simulink model "conSys_2robots_2_vR2014a"  (Simulink 8.3)
settings: Solver=FixedStepDiscrete  StartTime=0.0  StopTime=200  FixedStep=Ts  RelTol=1e-3
values from neighbouring files (symbols this model uses):
  ck = double(max(abs([par.q0_r1;par.q0_r2] - [par.q0r_r1;par.q0r_r2]))*20/7000 + 6)    [startUp_conSys_2robots_1_vGPU_vR2014a.m]    (also in startUp_conSys_2robots_1_vR2014a.m = max(abs([par.q0_r1;par.q0_r2] - [par.q0r_r1;par.q0r_r2]))*20; startUp_conSys_2robots_2_vR2014a.m = max(abs([par.q0_r1;par.q0_r2] - [par.q0r_r1;par.q0r_r2]))*20; startUp_conSys_2robots_3_vR2014a.m = max(abs([par.q0_r1;par.q0_r2] - [par.q0r_r1;par.q0r_r2]))*20; startUp_conSys_2robots_4_vR2014a.m = max(abs([par.q0_r1;par.q0_r2] - [par.q0r_r1;par.q0r_r2]))*20)
  d_0 = 2000    [startUp_conSys_2robots_1_vGPU_vR2014a.m]    (also in startUp_conSys_2robots_1_vR2014a.m = 200; startUp_conSys_2robots_2_vR2014a.m = 200; startUp_conSys_2robots_3_vR2014a.m; startUp_conSys_2robots_4_vR2014a.m = 200)
  do1r_0 = dthc_0 + dph1_0    (= 0.2)    [startUp_conSys_2robots_1_vGPU_vR2014a.m]    (also in startUp_conSys_2robots_1_vR2014a.m = 0; startUp_conSys_2robots_2_vR2014a.m = 0; startUp_conSys_2robots_3_vR2014a.m = 0; startUp_conSys_2robots_4_vR2014a.m = 0)
  do2r_0 = dthc_0 + dph2_0    (= -0.2)    [startUp_conSys_2robots_1_vGPU_vR2014a.m]    (also in startUp_conSys_2robots_1_vR2014a.m = 0; startUp_conSys_2robots_2_vR2014a.m = 0; startUp_conSys_2robots_3_vR2014a.m = 0; startUp_conSys_2robots_4_vR2014a.m = 0)
  dx1r_0 = dxc_0 + sin(thc_0)*dd_0 + d_0*cos(thc_0)*dthc_0    [startUp_conSys_2robots_1_vGPU_vR2014a.m]    (also in startUp_conSys_2robots_1_vR2014a.m; startUp_conSys_2robots_2_vR2014a.m; startUp_conSys_2robots_3_vR2014a.m; startUp_conSys_2robots_4_vR2014a.m)
  dx2r_0 = dxc_0 - sin(thc_0)*dd_0 - d_0*cos(thc_0)*dthc_0    [startUp_conSys_2robots_1_vGPU_vR2014a.m]    (also in startUp_conSys_2robots_1_vR2014a.m; startUp_conSys_2robots_2_vR2014a.m; startUp_conSys_2robots_3_vR2014a.m; startUp_conSys_2robots_4_vR2014a.m)
  dy1r_0 = dyc_0 + cos(thc_0)*dd_0 - d_0*sin(thc_0)*dthc_0    [startUp_conSys_2robots_1_vGPU_vR2014a.m]    (also in startUp_conSys_2robots_1_vR2014a.m; startUp_conSys_2robots_2_vR2014a.m; startUp_conSys_2robots_3_vR2014a.m; startUp_conSys_2robots_4_vR2014a.m)
  dy2r_0 = dyc_0 - cos(thc_0)*dd_0 + d_0*sin(thc_0)*dthc_0    [startUp_conSys_2robots_1_vGPU_vR2014a.m]    (also in startUp_conSys_2robots_1_vR2014a.m; startUp_conSys_2robots_2_vR2014a.m; startUp_conSys_2robots_3_vR2014a.m; startUp_conSys_2robots_4_vR2014a.m)
  o1r_0 = pi/2 - thc_0    (= 0)    [startUp_conSys_2robots_1_vGPU_vR2014a.m]    (also in startUp_conSys_2robots_1_vR2014a.m = pi/2 - thc_0; startUp_conSys_2robots_2_vR2014a.m = pi/2 - thc_0; startUp_conSys_2robots_3_vR2014a.m; startUp_conSys_2robots_4_vR2014a.m = th1_0)
  o2r_0 = pi/2 - thc_0    (= 0)    [startUp_conSys_2robots_1_vGPU_vR2014a.m]    (also in startUp_conSys_2robots_1_vR2014a.m = pi/2 - thc_0; startUp_conSys_2robots_2_vR2014a.m = pi/2 - thc_0; startUp_conSys_2robots_3_vR2014a.m; startUp_conSys_2robots_4_vR2014a.m = th2_0)
  thc_0 = pi/2    (= 1.57079632679)    [startUp_conSys_2robots_1_vGPU_vR2014a.m]    (also in startUp_conSys_2robots_1_vR2014a.m = atan2(1/25,1/12.5) + pi/2; startUp_conSys_2robots_2_vR2014a.m = atan2(1/25,1/12.5) + pi/2; startUp_conSys_2robots_3_vR2014a.m; startUp_conSys_2robots_4_vR2014a.m = atan2(1/25,1/12.5) + pi/2)
  Ts = 1/200    (= 0.005)    [startUp_conSys_2robots_1_vGPU_vR2014a.m]    (also in startUp_conSys_2robots_1_vR2014a.m = 0.0125; startUp_conSys_2robots_2_vR2014a.m = 0.01; startUp_conSys_2robots_3_vR2014a.m; startUp_conSys_2robots_4_vR2014a.m)
  x1_0 = 12000    [startUp_conSys_2robots_1_vGPU_vR2014a.m]    (also in startUp_conSys_2robots_1_vR2014a.m = 13178.9; startUp_conSys_2robots_2_vR2014a.m = 13178.9; startUp_conSys_2robots_3_vR2014a.m; startUp_conSys_2robots_4_vR2014a.m = 13178.9)
  x2_0 = 8000    [startUp_conSys_2robots_1_vGPU_vR2014a.m]    (also in startUp_conSys_2robots_1_vR2014a.m = 12821.1; startUp_conSys_2robots_2_vR2014a.m = 12821.1; startUp_conSys_2robots_3_vR2014a.m; startUp_conSys_2robots_4_vR2014a.m = 12821.1)
  xc_0 = 10000    [startUp_conSys_2robots_1_vGPU_vR2014a.m]    (also in startUp_conSys_2robots_1_vR2014a.m = 13000; startUp_conSys_2robots_2_vR2014a.m = 13000; startUp_conSys_2robots_3_vR2014a.m; startUp_conSys_2robots_4_vR2014a.m = 13000)
  y1_0 = 10000    [startUp_conSys_2robots_1_vGPU_vR2014a.m]    (also in startUp_conSys_2robots_1_vR2014a.m = 12910.6; startUp_conSys_2robots_2_vR2014a.m = 12910.6; startUp_conSys_2robots_3_vR2014a.m; startUp_conSys_2robots_4_vR2014a.m = 12910.6)
  y2_0 = 10000    [startUp_conSys_2robots_1_vGPU_vR2014a.m]    (also in startUp_conSys_2robots_1_vR2014a.m = 13089.4; startUp_conSys_2robots_2_vR2014a.m = 13089.4; startUp_conSys_2robots_3_vR2014a.m; startUp_conSys_2robots_4_vR2014a.m = 13089.4)
  yc_0 = 10000    [startUp_conSys_2robots_1_vGPU_vR2014a.m]    (also in startUp_conSys_2robots_1_vR2014a.m = 13000; startUp_conSys_2robots_2_vR2014a.m = 13000; startUp_conSys_2robots_3_vR2014a.m; startUp_conSys_2robots_4_vR2014a.m = 13000)
undefined symbols (not defined in the file or in its folder): absoluteAngle01_vR2014a, absoluteAngle02_vR2014a, absoluteAngle03_vR2014a, absoluteAngle04_vR2014a, absoluteAngle05_vR2014a, absoluteAngle06_vR2014a, absoluteAngle07_vR2014a, DiscIntNeverNeededParam
undefined symbols (not defined in the file): ADAMS_cwd, ADAMS_exec, ADAMS_host, ADAMS_init, ADAMS_inputs, ADAMS_outputs, ADAMS_prefix, ADAMS_static, ADAMS_sysdir
libraries: simulink x18, cstblocks x1
(part 2 of 2)

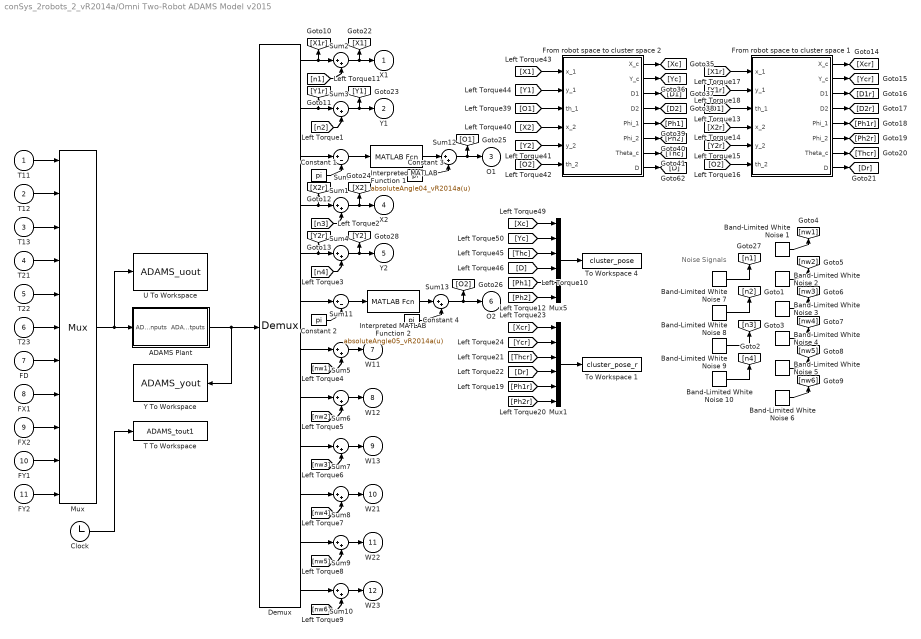
== system conSys_2robots_2_vR2014a/Omni Two-Robot ADAMS Model v2015 ==
  note: Noise Signals
  T11 : Inport
  T12 : Inport  Port=2
  T13 : Inport  Port=3
  T21 : Inport  Port=4
  T22 : Inport  Port=5
  T23 : Inport  Port=6
  FD : Inport  Port=7
  FX1 : Inport  Port=8
  FX2 : Inport  Port=9
  FY1 : Inport  Port=10
  FY2 : Inport  Port=11
  ADAMS Plant : Subsystem  LoadFcn=|  InitFcn=clear mex  mask(Adams Plant){exevie=ADAMS_sysdir, nam_in=ADAMS_inputs, namout=ADAMS_outputs, nampre=ADAMS_prefix, outfil=ADAMS_prefix, exesol=ADAMS_exec, stat=ADAMS_static, inicmd=[ADAMS_init], exetyp=C++, comtyp=PIPE(DDE), workdir=ADAMS_cwd, ada_host=ADAMS_host, modani=batch, modsim=discrete, dft=no, simulink_lead_cosim=yes, pin_interp_order=0, pout_extrap_order=0, pin_extrap_order=0, pout_interp_order=0, dt_out=Ts, o_rate=1, more=off}
      | %check based on dialog box setting for when setting by popup menu                                             
      | if exist('ADAMS_solver_type')                                                                                 
      |   if strcmp(ADAMS_solver_type,'C++')                                                                          
      |     set_param(gcb,'exetyp','C++');                                                                            
      |   else                                                                                                        
      |     set_param(gcb,'exetyp','Fortran');                                                                        
      |   end                                                                                                         
      | else                                                                                                          
      |   set_param(gcb,'exetyp','C++');                                                                              
      | end                                                                                                           
      | %set the mode if using acar_solver                                                                            
      | %REQUIRED HERE BECAUSE BELOW CAUSES MDLTERMINATE TO BE CALLED 2 TIMES IN MIDDLE OF SIMULATION WHEN SET IN MASK
      |                                                                                                               
      | %enable the direct feedthrough, sim mode, anim mode parameters by default                                     
      |                                                                                                               
      | if exist('set_some_params_states')                                                                            
      |                                                                                                               
      |   set_some_params_states({'dft','modsim','modani'},{'on','on','on'},'MaskEnables',gcb)                        
      |   %turn on direct feedthrough option                                                                          
      |   set_some_params_states({'dft'},{'on'},'MaskVisibilities',gcb)                                               
      |                                                                                                               
      |  end                                                                                                          
      |                                                                                                               
      |                                                                                                               
      | if exist('ADAMS_exec')                                                                                        
      |   if and(strcmp(get_param(gcb,'exesol'),'ADAMS_exec'),strcmp(ADAMS_exec,'acar_solver'))                       
      |     %set the sim mode to discrete -- only supported mode                                                      
      |     set_param(gcb,'modsim','discrete')                                                                        
      |      %turn off direct feedthrough option                                                                      
      |      set_some_params_states({'dft'},{'off'},'MaskVisibilities',gcb)                                           
      |     %set the animation mode to batch -- only supported mode                                                   
      |     set_param(gcb,'modani','batch')                                                                           
      |     %disable the direct feedthrough, sim mode, anim mode parameters                                           
      |     set_some_params_states({'modsim','modani'},{'off','off'},'MaskEnables',gcb)                               
      |   end                                                                                                         
      | end
      mask prompts: exevie "Adams install directory"; nam_in "Adams/View input names"; namout "Adams/View output names"; nampre "Adams model file prefix"; outfil "Output files prefix (opt.: if blank - no output)"; exesol "User executable (opt.: if blank - use standard)"; stat "Initial static simulation flag"; inicmd "Initialization commands"; exetyp "Adams/Solver type"; comtyp "Interprocess option"; workdir "Adams working directory"; ada_host "Adams host"; modani "Animation mode"; modsim "Simulation mode"; dft "Direct feedthrough"; simulink_lead_cosim "Discrete Computational Order - Simulink Leads Adams"; pin_interp_order "Plant input interpolation order"; pout_extrap_order "Plant output extrapolation order"; pin_extrap_order "Plant input extrapolation order"; pout_interp_order "Plant output interpolation order"; dt_out "Communication interval"; o_rate "Number of communications per output step"; more "More parameters"
      mask help: Simulate any Adams plant model either in Adams/Solver form (.adm file) or in Adams/View form (.cmd file)
      settings: OpenFcn=|
      | open_system(gcb,'mask')
      | if not(exist('set_some_params_states'))
      | 
      | warning('The script "set_some_params_states.m" cannot be found in the MATLAB PATH.  Cannot update the ADAMS Plant S-Function parameters.')
      | 
      | warning('Recommended action(optional):  run the Adams/Controls .m file first to help choose the correct settings in the Adams S-Function block.')
      | 
      | end
      mask Help:
      | <html>
      | This S-Function represents the non-linear Adams Plant with the inputs sent to the Adams model <br>
      |  and the outputs generated by the Adams model.  See the Adams/Controls documentation for more <br>
      | information.  This plant uses the following variables:<br>
      | <br>
      | <b>ADAMS_sysdir  :</b> Adams installation directory<br>
      | <b>ADAMS_inputs  :</b> Input variables View names vector<br>
      | <b>ADAMS_outputs :</b> Outputs variables View names vector<br>
      | <b>ADAMS_prefix  : </b>ADAMS model files prefix (.adm, .cmd); also doubles as output files prefix<br>
      | <b>ADAMS_exec :</b> Adams/Solver user library or keyword (e.g., acar_solver)<br>
      | <b>ADAMS_static :</b> yes|no - initial static before Co-simulation(discrete)/Function Evaluation(continuous)<br>
      | <b>ADAMS_init :</b>Initialization commands (i.e., Adams/View or Solver commands, depending on setting for Animation mode)<br>
      | <b>ADAMS_cwd : </b> Current working directory (for TCP/IP)<br>
      | <b>ADAMS_host : </b>Name of Adams server host (for TCP/IP)<br>
      | <b>ADAMS_mode :</b> Linear or non-linear (i.e., co-sim, function eval)<br>
      | <b>ADAMS_solver_type :</b>Fortran or C++ (used to set popup menu when first loaded) <br>
      | 
      | 
      | <br>
      | The following settings can be chosen:<br>
      | <br>
      | <b>Adams/Solver type:</b>  Fortran or C++ (will also set ADAMS_solver_type)<br>
      | <b>Interprocess option:</b> Pipe(DDE) or TCP/IP; TCP/IP can allow different machines run Adams and MATLAB<br>
      | <b>Animation mode:</b> batch (Solver, uses .adm) or interactive (View, uses .cmd)<br>
      | <b>Simulation mode:</b> discrete (Co-simulation) or continuous (Function Evaluation)<br>
      | <b>Discrete Computational Order - Simulink Lead Adams:</b> for discrete mode, chooses if Simulink leads the integration (yes) or lags (no);<br> if set to "no", can remove algebraic loop<br>
      | <b>Plant input interpolation order:</b> 0 = zero-order hold; 1 = linear (discrete mode only, where Simulink leads)<br>
      | <b>Plant output extrapolation order:</b> 0 = zero-order hold;1 = linear(discrete mode only, where Simulink leads)<br>
      | <b>Plant input extrapolation order:</b> 0 = zero-order hold; 1 = linear (discrete mode only, where Adams leads)<br>
      | <b>Plant output interpolation order:</b> 0 = zero-order hold;1 = linear(discrete mode only, where Adams leads)<br>
      | <b>Direct feedthrough:</b> yes|no - yes = Input directly effect output(continuous mode-only)<br>
      | <b>Communication interval:</b> Time step at which Co-simulation exchange information (e.g.,0.005); also controls <br>output for continuous mode (Function Evaluation)<br>
      | <b>Number of communications per output step: </b>Sets Adams output rate (.res, .req, .gra) integer value (default: 1)<br>
      | </html>
      mask Callback exesol:
      | if exist('set_some_params_states')
      | %enable the direct feedthrough, sim mode, anim mode parameters
      | set_some_params_states({'dft','modsim','modani'},{'on','on','on'},'MaskEnables',gcb)
      | %turn on direct feedthrough option
      | set_some_params_states({'dft'},{'on'},'MaskVisibilities',gcb)
      | end
      | 
      | if exist('ADAMS_exec')
      |   if and(strcmp(get_param(gcb,'exesol'),'ADAMS_exec'),strcmp(ADAMS_exec,'acar_solver'))
      |     %set the sim mode to discrete -- only supported mode
      |     %REMOVED:  BELOW CAUSES MDLTERMINATE TO BE CALLED 2 TIMES IN MIDDLE OF SIMULATION
      |     %Now in LoadFcn callback
      |     %set_param(gcb,'modsim','discrete')
      |      %turn off direct feedthrough option
      |     set_some_params_states({'dft'},{'off'},'MaskVisibilities',gcb)
      |     %set the animation mode to batch -- only supported mode
      |     %REMOVED:  BELOW CAUSES MDLTERMINATE TO BE CALLED 2 TIMES IN MIDDLE OF SIMULATION
      |     %Now in LoadFcn callback
      |     %set_param(gcb,'modani','batch')
      |     %disable the direct feedthrough, sim mode, anim mode parameters
      |     set_some_params_states({'modsim','modani'},{'off','off'},'MaskEnables',gcb)
      |   end
      | end
      mask TypeOptions exetyp: Fortran | C++
      mask Callback exetyp:
      | if strcmp(get_param(gcb,'exetyp'),'C++')
      |     ADAMS_solver_type='C++';
      | else
      |     ADAMS_solver_type='Fortran';
      | end
      mask TypeOptions comtyp: PIPE(DDE) | TCP/IP
      mask Callback comtyp:
      | if exist('set_some_params_states')
      | if strcmp(get_param(gcb,'comtyp'),'PIPE(DDE)')
      |     %turn off cwd, host options
      |     set_some_params_states({'ada_host','workdir'},{'off','off'},'MaskVisibilities',gcb)
      | else%if strcmp(get_param(gcb,'modsim'),'TCP/IP')
      |     %turn on cwd, host options
      |     set_some_params_states({'ada_host','workdir'},{'on','on'},'MaskVisibilities',gcb)
      | end
      | end
      mask TypeOptions modani: batch | interactive
      mask TypeOptions modsim: discrete | continuous
      mask Callback modsim:
      | if exist('set_some_params_states')
      | if strcmp(get_param(gcb,'modsim'),'discrete')
      |      %turn off direct feedthrough option
      |     set_some_params_states({'dft'},{'off'},'MaskVisibilities',gcb)
      |     %turn on discrete co-sim type if want to see more
      |     if strcmp(get_param(gcb,'more'),'on')
      |         set_some_params_states({'simulink_lead_cosim'},{'on'},'MaskVisibilities',gcb)
      |     end
      |     if strcmp(get_param(gcb,'simulink_lead_cosim'),'yes')
      |         %turn on interpolation/extrapolation options
      |         set_some_params_states({'pin_interp_order','pout_extrap_order',},{'on','on'},'MaskVisibilities',gcb)
      |     else
      |         set_some_params_states({'pin_extrap_order','pout_interp_order'},{'on','on'},'MaskVisibilities',gcb)
      |     end
      | else%if strcmp(get_param(gcb,'modsim'),'continuous')
      |      %turn off direct feedthrough option
      |     set_some_params_states({'dft'},{'on'},'MaskVisibilities',gcb)
      |     %turn off interpolation/extrapolation options
      |     set_some_params_states({'pin_interp_order','pout_extrap_order','pin_extrap_order','pout_interp_order','simulink_lead_cosim'},{'off','off','off','off','off'},'MaskVisibilities',gcb)
      | end
      | end
      mask TypeOptions dft: no | yes
      mask TypeOptions simulink_lead_cosim: yes | no
      mask Callback simulink_lead_cosim:
      | if exist('set_some_params_states')
      | if (strcmp(get_param(gcb,'simulink_lead_cosim'),'yes') && strcmp(get_param(gcb,'modsim'),'discrete'))
      |      %turn off unused interpolate/extrapolate options
      |     set_some_params_states({'pin_extrap_order','pout_interp_order'},{'off','off'},'MaskVisibilities',gcb)
      |     %turn on used interpolate/extrapolate options
      |     set_some_params_states({'pin_interp_order','pout_extrap_order'},{'on','on'},'MaskVisibilities',gcb)
      | elseif (strcmp(get_param(gcb,'simulink_lead_cosim'),'no') && strcmp(get_param(gcb,'modsim'),'discrete'))
      |     %turn on used interpolate/extrapolate options
      |     set_some_params_states({'pin_extrap_order','pout_interp_order'},{'on','on'},'MaskVisibilities',gcb)
      |      %turn off unused interpolate/extrapolate options
      |     set_some_params_states({'pin_interp_order','pout_extrap_order'},{'off','off'},'MaskVisibilities',gcb)
      | end
      | end
      mask TypeOptions pin_interp_order: 0 | 1
      mask TypeOptions pout_extrap_order: 0 | 1
      mask TypeOptions pin_extrap_order: 0 | 1
      mask TypeOptions pout_interp_order: 0 | 1
      mask Callback more:
      | if exist('set_some_params_states')
      | if (strcmp(get_param(gcb,'more'),'on'))
      |      %turn on infrequently used options
      |     set_some_params_states({'exevie','nam_in','namout','exesol','stat','inicmd'},{'on','on','on','on','on','on'},'MaskVisibilities',gcb)
      |     if strcmp(get_param(gcb,'modsim'),'discrete')
      |         set_some_params_states({'simulink_lead_cosim'},{'on'},'MaskVisibilities',gcb)
      |     end
      | elseif (strcmp(get_param(gcb,'more'),'off'))
      |     %turn off infrequently used options
      |     set_some_params_states({'exevie','nam_in','namout','exesol','stat','inicmd'},{'off','off','off','off','off','off'},'MaskVisibilities',gcb)
      |     if strcmp(get_param(gcb,'modsim'),'discrete')
      |         set_some_params_states({'simulink_lead_cosim'},{'off'},'MaskVisibilities',gcb)
      |     end
      | end
      | end
      mask Display: disp( 'MSC Software' )
  Band-Limited White Noise {1..6} (6 alike) : simulink/Sources/Band-Limited White Noise  Cov=[0.001]  Ts=Ts  seed=[23341]
  Band-Limited White Noise {7..10} (4 alike) : simulink/Sources/Band-Limited White Noise  Cov=[0.4]  Ts=Ts  seed=[23341]
  Clock : Clock
  Constant {1..4} (4 alike) : Constant  Value=pi
  Demux : Demux  Outputs=12
  From robot space to cluster space 1 : Subsystem
  From robot space to cluster space 2 : Subsystem
  Interpreted MATLAB Function 1 : MATLABFcn  MATLABFcn=absoluteAngle04_vR2014a(u)
  Interpreted MATLAB Function 2 : MATLABFcn  MATLABFcn=absoluteAngle05_vR2014a(u)
  Mux : Mux  Inputs=11
  Mux1 : Mux  Inputs=6
  Mux5 : Mux  Inputs=6
  Sum : Sum  Inputs=|+-
  Sum{1..10,12..13} (12 alike) : Sum  Inputs=|++
  Sum11 : Sum  Inputs=|+-
  T To Workspace : ToWorkspace  VariableName=ADAMS_tout1
      settings: MaxDataPoints=100000
  To Workspace 1 : ToWorkspace  VariableName=cluster_pose_r  SaveFormat=Structure With Time  SampleTime=-1
  To Workspace 4 : ToWorkspace  VariableName=cluster_pose  SaveFormat=Structure With Time  SampleTime=-1
  U To Workspace : ToWorkspace  VariableName=ADAMS_uout
      settings: MaxDataPoints=100000
  Y To Workspace : ToWorkspace  VariableName=ADAMS_yout
      settings: MaxDataPoints=100000
  X1 : Outport
  Y1 : Outport  Port=2
  O1 : Outport  Port=3
  X2 : Outport  Port=4
  Y2 : Outport  Port=5
  O2 : Outport  Port=6
  W11 : Outport  Port=7
  W12 : Outport  Port=8
  W13 : Outport  Port=9
  W21 : Outport  Port=10
  W22 : Outport  Port=11
  W23 : Outport  Port=12
  wires:
  T11/1 -> Mux/1
  T12/1 -> Mux/2
  T13/1 -> Mux/3
  T21/1 -> Mux/4
  T22/1 -> Mux/5
  T23/1 -> Mux/6
  FD/1 -> Mux/7
  FX1/1 -> Mux/8
  FX2/1 -> Mux/9
  FY1/1 -> Mux/10
  FY2/1 -> Mux/11
  Band-Limited White Noise 7/1 -> [n1]
  Demux/1 -> Sum2/1, [X1r]
  Demux/2 -> [Y1r], Sum3/1
  Sum2/1 -> [X1], X1/1
  Sum3/1 -> [Y1], Y1/1
  Band-Limited White Noise 8/1 -> [n2]
  Band-Limited White Noise 9/1 -> [n3]
  Band-Limited White Noise 10/1 -> [n4]
  Demux/4 -> [X2r], Sum1/1
  Demux/5 -> [Y2r], Sum4/1
  Sum1/1 -> X2/1, [X2]
  Sum4/1 -> Y2/1, [Y2]
  [n1] -> Sum2/2
  [n2] -> Sum3/2
  [n3] -> Sum1/2
  [n4] -> Sum4/2
  Band-Limited White Noise 1/1 -> [nw1]
  Band-Limited White Noise 2/1 -> [nw2]
  Band-Limited White Noise 3/1 -> [nw3]
  Band-Limited White Noise 4/1 -> [nw4]
  Band-Limited White Noise 5/1 -> [nw5]
  Band-Limited White Noise 6/1 -> [nw6]
  [nw1] -> Sum5/2
  [nw2] -> Sum6/2
  [nw3] -> Sum7/2
  [nw4] -> Sum8/2
  [nw5] -> Sum9/2
  [nw6] -> Sum10/2
  Demux/7 -> Sum5/1
  Sum5/1 -> W11/1
  Demux/8 -> Sum6/1
  Sum6/1 -> W12/1
  Demux/9 -> Sum7/1
  Sum7/1 -> W13/1
  Demux/10 -> Sum8/1
  Sum8/1 -> W21/1
  Demux/11 -> Sum9/1
  Sum9/1 -> W22/1
  Demux/12 -> Sum10/1
  Sum10/1 -> W23/1
  Demux/3 -> Sum/1
  Constant 1/1 -> Sum/2
  Sum/1 -> Interpreted MATLAB Function 1/1
  Demux/6 -> Sum11/1
  Constant 2/1 -> Sum11/2
  Sum11/1 -> Interpreted MATLAB Function 2/1
  Interpreted MATLAB Function 1/1 -> Sum12/1
  Sum12/1 -> [O1], O1/1
  Constant 3/1 -> Sum12/2
  Interpreted MATLAB Function 2/1 -> Sum13/1
  Sum13/1 -> [O2], O2/1
  Constant 4/1 -> Sum13/2
  From robot space to cluster space 2/8(D) -> [D]
  From robot space to cluster space 2/7(Theta_c) -> [Thc]
  From robot space to cluster space 2/6(Phi_2) -> [Ph2]
  From robot space to cluster space 2/5(Phi_1) -> [Ph1]
  From robot space to cluster space 2/4(D2) -> [D2]
  From robot space to cluster space 2/3(D1) -> [D1]
  From robot space to cluster space 2/2(Y_c) -> [Yc]
  From robot space to cluster space 2/1(X_c) -> [Xc]
  [X1] -> From robot space to cluster space 2/1(x_1)
  [Y1] -> From robot space to cluster space 2/2(y_1)
  [O1] -> From robot space to cluster space 2/3(th_1)
  [X2] -> From robot space to cluster space 2/4(x_2)
  [Y2] -> From robot space to cluster space 2/5(y_2)
  [O2] -> From robot space to cluster space 2/6(th_2)
  [Thc] -> Mux5/3
  [D] -> Mux5/4
  [Xc] -> Mux5/1
  [Yc] -> Mux5/2
  Mux5/1 -> To Workspace 4/1
  [Ph1] -> Mux5/5
  [Ph2] -> Mux5/6
  From robot space to cluster space 1/8(D) -> [Dr]
  From robot space to cluster space 1/7(Theta_c) -> [Thcr]
  From robot space to cluster space 1/6(Phi_2) -> [Ph2r]
  From robot space to cluster space 1/5(Phi_1) -> [Ph1r]
  From robot space to cluster space 1/4(D2) -> [D2r]
  From robot space to cluster space 1/3(D1) -> [D1r]
  From robot space to cluster space 1/2(Y_c) -> [Ycr]
  From robot space to cluster space 1/1(X_c) -> [Xcr]
  [X1r] -> From robot space to cluster space 1/1(x_1)
  [Y1r] -> From robot space to cluster space 1/2(y_1)
  [O1] -> From robot space to cluster space 1/3(th_1)
  [X2r] -> From robot space to cluster space 1/4(x_2)
  [Y2r] -> From robot space to cluster space 1/5(y_2)
  [O2] -> From robot space to cluster space 1/6(th_2)
  [Thcr] -> Mux1/3
  [Dr] -> Mux1/4
  [Xcr] -> Mux1/1
  [Ycr] -> Mux1/2
  Mux1/1 -> To Workspace 1/1
  [Ph1r] -> Mux1/5
  [Ph2r] -> Mux1/6
  Clock/1 -> T To Workspace/1
  Mux/1 -> U To Workspace/1, ADAMS Plant/1(ADAMS inputs)
  ADAMS Plant/1(ADAMS outputs) -> Y To Workspace/1, Demux/1

== system conSys_2robots_2_vR2014a/Cluster Space Controller/Clutch 1 ==
  Input : Inport
  Constant1 : Constant  Value=2
  Digital Clock : DigitalClock  SampleTime=Ts
  Gain 1 : Gain  Gain=.5
  Product : Product
  Rear Wheel Angular Speed5 : Scope
      settings: YMin=0  YMax=2  SaveName=ScopeData5
  Sine Wave1 : Sin  Bias=1  Frequency=(pi/ck)  Phase=-pi/2  SampleTime=Ts
  Switch : Switch  Threshold=ck
  To Workspace 2 : ToWorkspace  VariableName=clutch  SaveFormat=Structure With Time  SampleTime=-1
  Output : Outport
  wires:
  Constant1/1 -> Switch/1
  Digital Clock/1 -> Switch/2
  Switch/1 -> Gain 1/1
  Input/1 -> Product/2
  Product/1 -> Output/1
  Sine Wave1/1 -> Switch/3
  Gain 1/1 -> To Workspace 2/1, Rear Wheel Angular Speed5/1, Product/1

== system conSys_2robots_2_vR2014a/Cluster Space Controller/Clutch 2 ==
  Input : Inport
  Constant1 : Constant  Value=2
  Digital Clock : DigitalClock  SampleTime=Ts
  Gain 1 : Gain  Gain=.5
  Product : Product
  Rear Wheel Angular Speed5 : Scope
      settings: YMin=0  YMax=2  SaveName=ScopeData5
  Sine Wave1 : Sin  Bias=1  Frequency=(pi/ck)  Phase=-pi/2  SampleTime=Ts
  Switch : Switch  Threshold=ck
  Output : Outport
  wires:
  Gain 1/1 -> Product/1, Rear Wheel Angular Speed5/1
  Sine Wave1/1 -> Switch/3
  Product/1 -> Output/1
  Input/1 -> Product/2
  Switch/1 -> Gain 1/1
  Digital Clock/1 -> Switch/2
  Constant1/1 -> Switch/1

== system conSys_2robots_2_vR2014a/Cluster Space Controller/Clutch 3 ==
  Input : Inport
  Constant1 : Constant  Value=2
  Digital Clock : DigitalClock  SampleTime=Ts
  Gain 1 : Gain  Gain=.5
  Product : Product
  Rear Wheel Angular Speed5 : Scope
      settings: YMin=0  YMax=2  SaveName=ScopeData5
  Sine Wave1 : Sin  Bias=1  Frequency=(pi/ck)  Phase=-pi/2  SampleTime=Ts
  Switch : Switch  Threshold=ck
  Output : Outport
  wires:
  Constant1/1 -> Switch/1
  Digital Clock/1 -> Switch/2
  Switch/1 -> Gain 1/1
  Input/1 -> Product/2
  Product/1 -> Output/1
  Sine Wave1/1 -> Switch/3
  Gain 1/1 -> Rear Wheel Angular Speed5/1, Product/1

== system conSys_2robots_2_vR2014a/Cluster Space Controller/Clutch 4 ==
  Input : Inport
  Constant1 : Constant  Value=2
  Digital Clock : DigitalClock  SampleTime=Ts
  Gain 1 : Gain  Gain=.5
  Product : Product
  Rear Wheel Angular Speed5 : Scope
      settings: YMin=0  YMax=2  SaveName=ScopeData5
  Sine Wave1 : Sin  Bias=1  Frequency=(pi/ck)  Phase=-pi/2  SampleTime=Ts
  Switch : Switch  Threshold=ck
  Output : Outport
  wires:
  Gain 1/1 -> Product/1, Rear Wheel Angular Speed5/1
  Sine Wave1/1 -> Switch/3
  Product/1 -> Output/1
  Input/1 -> Product/2
  Switch/1 -> Gain 1/1
  Digital Clock/1 -> Switch/2
  Constant1/1 -> Switch/1

== system conSys_2robots_2_vR2014a/Cluster Space Controller/Clutch 5 ==
  Input : Inport
  Constant1 : Constant  Value=2
  Digital Clock : DigitalClock  SampleTime=Ts
  Gain 1 : Gain  Gain=.5
  Product : Product
  Rear Wheel Angular Speed5 : Scope
      settings: YMin=0  YMax=2  SaveName=ScopeData5
  Sine Wave1 : Sin  Bias=1  Frequency=(pi/ck)  Phase=-pi/2  SampleTime=Ts
  Switch : Switch  Threshold=ck
  Output : Outport
  wires:
  Constant1/1 -> Switch/1
  Digital Clock/1 -> Switch/2
  Switch/1 -> Gain 1/1
  Input/1 -> Product/2
  Product/1 -> Output/1
  Sine Wave1/1 -> Switch/3
  Gain 1/1 -> Rear Wheel Angular Speed5/1, Product/1

== system conSys_2robots_2_vR2014a/Cluster Space Controller/Clutch 6 ==
  Input : Inport
  Constant1 : Constant  Value=2
  Digital Clock : DigitalClock  SampleTime=Ts
  Gain 1 : Gain  Gain=.5
  Product : Product
  Rear Wheel Angular Speed5 : Scope
      settings: YMin=0  YMax=2  SaveName=ScopeData5
  Sine Wave1 : Sin  Bias=1  Frequency=(pi/ck)  Phase=-pi/2  SampleTime=Ts
  Switch : Switch  Threshold=ck
  Output : Outport
  wires:
  Gain 1/1 -> Product/1, Rear Wheel Angular Speed5/1
  Sine Wave1/1 -> Switch/3
  Product/1 -> Output/1
  Input/1 -> Product/2
  Switch/1 -> Gain 1/1
  Digital Clock/1 -> Switch/2
  Constant1/1 -> Switch/1

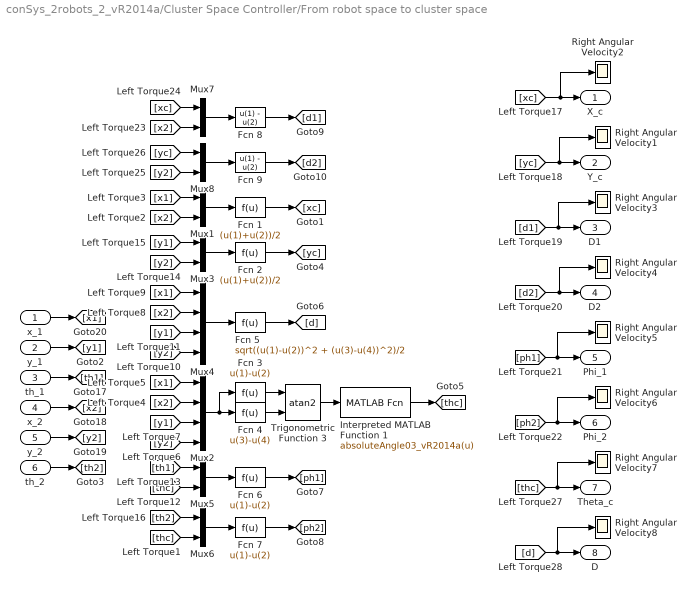
== system conSys_2robots_2_vR2014a/Cluster Space Controller/From robot space to cluster space ==
  x_1 : Inport
  y_1 : Inport  Port=2
  th_1 : Inport  Port=3
  x_2 : Inport  Port=4
  y_2 : Inport  Port=5
  th_2 : Inport  Port=6
  Fcn 1 : Fcn  Expr=(u(1)+u(2))/2
  Fcn 2 : Fcn  Expr=(u(1)+u(2))/2
  Fcn 3 : Fcn  Expr=u(1)-u(2)
  Fcn 4 : Fcn  Expr=u(3)-u(4)
  Fcn 5 : Fcn  Expr=sqrt((u(1)-u(2))^2 + (u(3)-u(4))^2)/2
  Fcn 6 : Fcn  Expr=u(1)-u(2)
  Fcn 7 : Fcn  Expr=u(1)-u(2)
  Fcn 8 : Fcn  Expr=u(1) - u(2)
  Fcn 9 : Fcn  Expr=u(1) - u(2)
  Interpreted MATLAB Function 1 : MATLABFcn  MATLABFcn=absoluteAngle03_vR2014a(u)  SampleTime=Ts
  Mux{1,3,5..8} (6 alike) : Mux  Inputs=2
  Mux2 : Mux
  Mux4 : Mux
  Right Angular Velocity{1..8} (8 alike) : Scope
      Right Angular Velocity1 settings: YMin=2400  YMax=2600  SaveName=ScopeData38
      Right Angular Velocity2 settings: YMin=2400  YMax=2600  SaveName=ScopeData36
      Right Angular Velocity3 settings: YMin=2400  YMax=2600  SaveName=ScopeData48
      Right Angular Velocity4 settings: YMin=0  YMax=700  SaveName=ScopeData49
      Right Angular Velocity5 settings: YMin=2400  YMax=2600  SaveName=ScopeData50
      Right Angular Velocity6 settings: YMin=2400  YMax=2600  SaveName=ScopeData51
      Right Angular Velocity7 settings: YMin=-10  YMax=10  SaveName=ScopeData80
      Right Angular Velocity8 settings: YMin=1350  YMax=1392.5  SaveName=ScopeData85
  Trigonometric Function 3 : Trigonometry  Operator=atan2
  X_c : Outport
  Y_c : Outport  Port=2
  D1 : Outport  Port=3
  D2 : Outport  Port=4
  Phi_1 : Outport  Port=5
  Phi_2 : Outport  Port=6
  Theta_c : Outport  Port=7
  D : Outport  Port=8
  wires:
  [d] -> D/1, Right Angular Velocity8/1
  [thc] -> Right Angular Velocity7/1, Theta_c/1
  Fcn 9/1 -> [d2]
  Mux8/1 -> Fcn 9/1
  [y2] -> Mux8/2
  [yc] -> Mux8/1
  Fcn 8/1 -> [d1]
  Mux7/1 -> Fcn 8/1
  [x2] -> Mux7/2
  [xc] -> Mux7/1
  Fcn 7/1 -> [ph2]
  Mux6/1 -> Fcn 7/1
  [thc] -> Mux6/2
  [th2] -> Mux6/1
  [y1] -> Mux2/3
  [y2] -> Mux2/4
  [x1] -> Mux2/1
  [x2] -> Mux2/2
  Fcn 2/1 -> [yc]
  Mux3/1 -> Fcn 2/1
  [y2] -> Mux3/2
  [y1] -> Mux3/1
  Fcn 1/1 -> [xc]
  Mux1/1 -> Fcn 1/1
  [x2] -> Mux1/2
  [x1] -> Mux1/1
  [ph2] -> Phi_2/1, Right Angular Velocity6/1
  [ph1] -> Phi_1/1, Right Angular Velocity5/1
  [d2] -> D2/1, Right Angular Velocity4/1
  [d1] -> D1/1, Right Angular Velocity3/1
  [yc] -> Y_c/1, Right Angular Velocity1/1
  [xc] -> X_c/1, Right Angular Velocity2/1
  Fcn 6/1 -> [ph1]
  Mux5/1 -> Fcn 6/1
  [thc] -> Mux5/2
  [th1] -> Mux5/1
  Fcn 5/1 -> [d]
  Mux4/1 -> Fcn 5/1
  [y1] -> Mux4/3
  [x2] -> Mux4/2
  [y2] -> Mux4/4
  [x1] -> Mux4/1
  Fcn 4/1 -> Trigonometric Function 3/2
  Fcn 3/1 -> Trigonometric Function 3/1
  Mux2/1 -> Fcn 4/1, Fcn 3/1
  Trigonometric Function 3/1 -> Interpreted MATLAB Function 1/1
  Interpreted MATLAB Function 1/1 -> [thc]
  th_2/1 -> [th2]
  x_1/1 -> [x1]
  y_1/1 -> [y1]
  th_1/1 -> [th1]
  x_2/1 -> [x2]
  y_2/1 -> [y2]

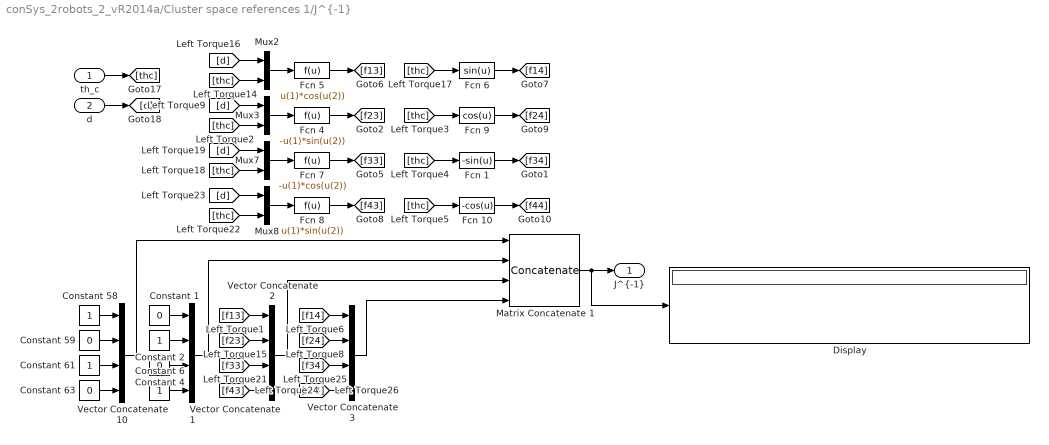
== system conSys_2robots_2_vR2014a/Cluster space references 1/J^{-1} ==
  th_c : Inport
  d : Inport  Port=2
  Constant {1,4,59,63} (4 alike) : Constant  Value=0
  Constant {2,6,58,61} (4 alike) : Constant
  Display : Display
  Fcn 1 : Fcn  Expr=-sin(u)
  Fcn 10 : Fcn  Expr=-cos(u)
  Fcn 4 : Fcn  Expr=-u(1)*sin(u(2))
  Fcn 5 : Fcn  Expr=u(1)*cos(u(2))
  Fcn 6 : Fcn  Expr=sin(u)
  Fcn 7 : Fcn  Expr=-u(1)*cos(u(2))
  Fcn 8 : Fcn  Expr=u(1)*sin(u(2))
  Fcn 9 : Fcn  Expr=cos(u)
  Matrix Concatenate 1 : Concatenate  NumInputs=4  Mode=Multidimensional array  ConcatenateDimension=2
  Mux{2..3,7..8} (4 alike) : Mux  Inputs=2
  Vector Concatenate {1..3,10} (4 alike) : Concatenate  NumInputs=4
  "J^{-1}" : Outport
  wires:
  d/1 -> [d]
  th_c/1 -> [thc]
  Matrix Concatenate 1/1 -> "J^{-1}"/1, Display/1
  Vector Concatenate 10/1 -> Matrix Concatenate 1/1
  Vector Concatenate 1/1 -> Matrix Concatenate 1/2
  Vector Concatenate 2/1 -> Matrix Concatenate 1/3
  Constant 58/1 -> Vector Concatenate 10/1
  Constant 59/1 -> Vector Concatenate 10/2
  Constant 61/1 -> Vector Concatenate 10/3
  Constant 63/1 -> Vector Concatenate 10/4
  Constant 1/1 -> Vector Concatenate 1/1
  Constant 2/1 -> Vector Concatenate 1/2
  Constant 4/1 -> Vector Concatenate 1/3
  Constant 6/1 -> Vector Concatenate 1/4
  Vector Concatenate 3/1 -> Matrix Concatenate 1/4
  [d] -> Mux2/1
  [thc] -> Mux2/2
  Mux2/1 -> Fcn 5/1
  Fcn 5/1 -> [f13]
  Fcn 6/1 -> [f14]
  [thc] -> Fcn 6/1
  [f13] -> Vector Concatenate 2/1
  [d] -> Mux3/1
  [thc] -> Mux3/2
  Mux3/1 -> Fcn 4/1
  Fcn 4/1 -> [f23]
  [f23] -> Vector Concatenate 2/2
  [d] -> Mux7/1
  [thc] -> Mux7/2
  Mux7/1 -> Fcn 7/1
  Fcn 7/1 -> [f33]
  [f33] -> Vector Concatenate 2/3
  [d] -> Mux8/1
  [thc] -> Mux8/2
  Mux8/1 -> Fcn 8/1
  Fcn 8/1 -> [f43]
  [f43] -> Vector Concatenate 2/4
  Fcn 9/1 -> [f24]
  [thc] -> Fcn 9/1
  Fcn 1/1 -> [f34]
  [thc] -> Fcn 1/1
  Fcn 10/1 -> [f44]
  [thc] -> Fcn 10/1
  [f14] -> Vector Concatenate 3/1
  [f24] -> Vector Concatenate 3/2
  [f34] -> Vector Concatenate 3/3
  [f44] -> Vector Concatenate 3/4

== system conSys_2robots_2_vR2014a/Cluster space references 1/Reference Variables ==
  Constant 1 : Constant  Value=0
  Constant 2 : Constant  Value=0
  Discrete-Time Integrator 1 : DiscreteIntegrator  IntegratorMethod=Integration: Trapezoidal  InitialCondition=do1r_0  SampleTime=Ts  ICPrevOutput=DiscIntNeverNeededParam  ICPrevScaledInput=DiscIntNeverNeededParam
  Discrete-Time Integrator 2 : DiscreteIntegrator  IntegratorMethod=Integration: Trapezoidal  InitialCondition=o1r_0  SampleTime=Ts  ICPrevOutput=DiscIntNeverNeededParam  ICPrevScaledInput=DiscIntNeverNeededParam
  Discrete-Time Integrator 3 : DiscreteIntegrator  IntegratorMethod=Integration: Trapezoidal  InitialCondition=do2r_0  SampleTime=Ts  ICPrevOutput=DiscIntNeverNeededParam  ICPrevScaledInput=DiscIntNeverNeededParam
  Discrete-Time Integrator 4 : DiscreteIntegrator  IntegratorMethod=Integration: Trapezoidal  InitialCondition=o2r_0  SampleTime=Ts  ICPrevOutput=DiscIntNeverNeededParam  ICPrevScaledInput=DiscIntNeverNeededParam
  Mux : Mux  Inputs=6
  Scope {1..4} (4 alike) : Scope
      Scope 1 settings: YMin=-0.45  YMax=0.47  SaveName=ScopeData18
      Scope 2 settings: YMin=-10  YMax=10  SaveName=ScopeData19
      Scope 3 settings: YMin=-0.45  YMax=0.47  SaveName=ScopeData27
      Scope 4 settings: YMin=-0.45  YMax=0.47  SaveName=ScopeData20
  Out : Outport  PortDimensions=6
  wires:
  Mux/1 -> Out/1
  [O1r] -> Mux/1
  [dO1r] -> Mux/2
  [dO2r] -> Mux/5
  [O2r] -> Mux/4
  [ddO1r] -> Mux/3
  [ddO2r] -> Mux/6
  Constant 2/1 -> Discrete-Time Integrator 1/1, [ddO1r]
  Discrete-Time Integrator 1/1 -> Discrete-Time Integrator 2/1, Scope 3/1, [dO1r]
  Discrete-Time Integrator 2/1 -> Scope 1/1, [O1r]
  Constant 1/1 -> [ddO2r], Discrete-Time Integrator 3/1
  Discrete-Time Integrator 3/1 -> [dO2r], Scope 4/1, Discrete-Time Integrator 4/1
  Discrete-Time Integrator 4/1 -> [O2r], Scope 2/1

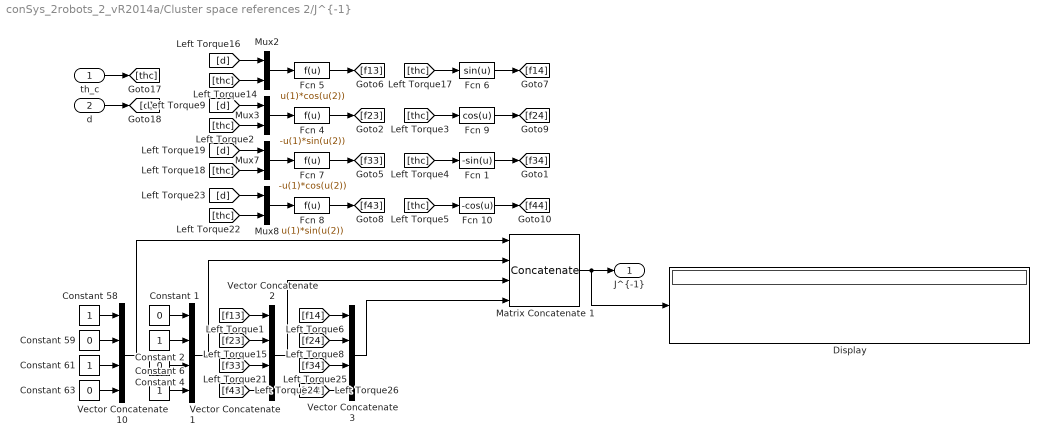
== system conSys_2robots_2_vR2014a/Cluster space references 2/J^{-1} ==
  th_c : Inport
  d : Inport  Port=2
  Constant {1,4,59,63} (4 alike) : Constant  Value=0
  Constant {2,6,58,61} (4 alike) : Constant
  Display : Display
  Fcn 1 : Fcn  Expr=-sin(u)
  Fcn 10 : Fcn  Expr=-cos(u)
  Fcn 4 : Fcn  Expr=-u(1)*sin(u(2))
  Fcn 5 : Fcn  Expr=u(1)*cos(u(2))
  Fcn 6 : Fcn  Expr=sin(u)
  Fcn 7 : Fcn  Expr=-u(1)*cos(u(2))
  Fcn 8 : Fcn  Expr=u(1)*sin(u(2))
  Fcn 9 : Fcn  Expr=cos(u)
  Matrix Concatenate 1 : Concatenate  NumInputs=4  Mode=Multidimensional array  ConcatenateDimension=2
  Mux{2..3,7..8} (4 alike) : Mux  Inputs=2
  Vector Concatenate {1..3,10} (4 alike) : Concatenate  NumInputs=4
  "J^{-1}" : Outport
  wires:
  [f44] -> Vector Concatenate 3/4
  [f34] -> Vector Concatenate 3/3
  [f24] -> Vector Concatenate 3/2
  [f14] -> Vector Concatenate 3/1
  [thc] -> Fcn 10/1
  Fcn 10/1 -> [f44]
  [thc] -> Fcn 1/1
  Fcn 1/1 -> [f34]
  [thc] -> Fcn 9/1
  Fcn 9/1 -> [f24]
  [f43] -> Vector Concatenate 2/4
  Fcn 8/1 -> [f43]
  Mux8/1 -> Fcn 8/1
  [thc] -> Mux8/2
  [d] -> Mux8/1
  [f33] -> Vector Concatenate 2/3
  Fcn 7/1 -> [f33]
  Mux7/1 -> Fcn 7/1
  [thc] -> Mux7/2
  [d] -> Mux7/1
  [f23] -> Vector Concatenate 2/2
  Fcn 4/1 -> [f23]
  Mux3/1 -> Fcn 4/1
  [thc] -> Mux3/2
  [d] -> Mux3/1
  [f13] -> Vector Concatenate 2/1
  [thc] -> Fcn 6/1
  Fcn 6/1 -> [f14]
  Fcn 5/1 -> [f13]
  Mux2/1 -> Fcn 5/1
  [thc] -> Mux2/2
  [d] -> Mux2/1
  Vector Concatenate 3/1 -> Matrix Concatenate 1/4
  Constant 6/1 -> Vector Concatenate 1/4
  Constant 4/1 -> Vector Concatenate 1/3
  Constant 2/1 -> Vector Concatenate 1/2
  Constant 1/1 -> Vector Concatenate 1/1
  Constant 63/1 -> Vector Concatenate 10/4
  Constant 61/1 -> Vector Concatenate 10/3
  Constant 59/1 -> Vector Concatenate 10/2
  Constant 58/1 -> Vector Concatenate 10/1
  Vector Concatenate 2/1 -> Matrix Concatenate 1/3
  Vector Concatenate 1/1 -> Matrix Concatenate 1/2
  Vector Concatenate 10/1 -> Matrix Concatenate 1/1
  Matrix Concatenate 1/1 -> Display/1, "J^{-1}"/1
  th_c/1 -> [thc]
  d/1 -> [d]

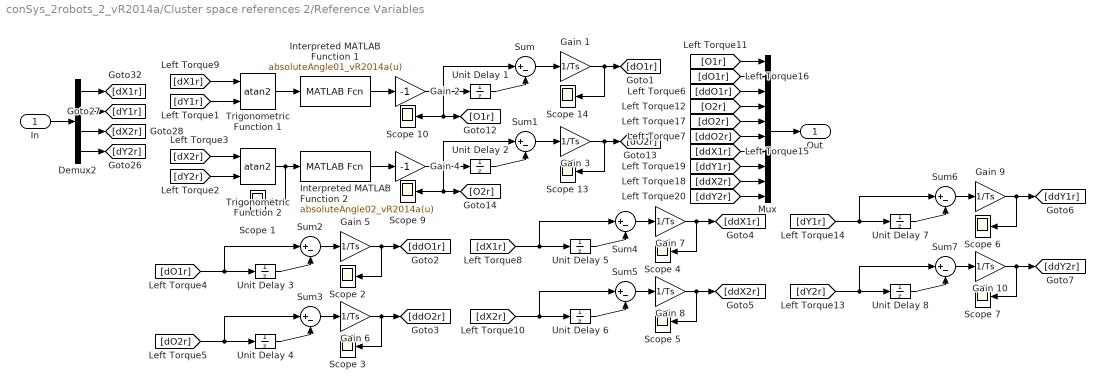
== system conSys_2robots_2_vR2014a/Cluster space references 2/Reference Variables ==
  In : Inport  PortDimensions=4
  Demux2 : Demux
  Gain {1,3,5..10} (8 alike) : Gain  Gain=1/Ts
  Gain 2 : Gain  Gain=-1
  Gain 4 : Gain  Gain=-1
  Interpreted MATLAB Function 1 : MATLABFcn  MATLABFcn=absoluteAngle01_vR2014a(u)
  Interpreted MATLAB Function 2 : MATLABFcn  MATLABFcn=absoluteAngle02_vR2014a(u)
  Mux : Mux  Inputs=10
  Scope {1..7,9..10,13..14} (11 alike) : Scope
      Scope 1 settings: YMin=0  YMax=10  SaveName=ScopeData61
      Scope 10 settings: TimeRange=500  YMin=-10  SaveName=ScopeData68
      Scope 13 settings: YMin=-0.45  YMax=0.47  SaveName=ScopeData71
      Scope 14 settings: YMin=-0.45  YMax=0.47  SaveName=ScopeData72
      Scope 2 settings: YMin=-0.02  YMax=0.02  SaveName=ScopeData26
      Scope 3 settings: YMin=-0.02  YMax=0.02  SaveName=ScopeData27
      Scope 4 settings: SaveName=ScopeData55
      Scope 5 settings: SaveName=ScopeData56
      Scope 6 settings: SaveName=ScopeData57
      Scope 7 settings: SaveName=ScopeData58
      Scope 9 settings: YMin=-10  YMax=10  SaveName=ScopeData67
  Sum{,1..7} (8 alike) : Sum  Inputs=|+-
  Trigonometric Function 1 : Trigonometry  Operator=atan2
  Trigonometric Function 2 : Trigonometry  Operator=atan2
  Unit Delay 1 : UnitDelay  InitialCondition=o1r_0  SampleTime=-1
  Unit Delay 2 : UnitDelay  InitialCondition=o2r_0  SampleTime=-1
  Unit Delay 3 : UnitDelay  InitialCondition=do1r_0  SampleTime=-1
  Unit Delay 4 : UnitDelay  InitialCondition=do2r_0  SampleTime=-1
  Unit Delay 5 : UnitDelay  InitialCondition=dx1r_0  SampleTime=-1
  Unit Delay 6 : UnitDelay  InitialCondition=dx2r_0  SampleTime=-1
  Unit Delay 7 : UnitDelay  InitialCondition=dy1r_0  SampleTime=-1
  Unit Delay 8 : UnitDelay  InitialCondition=dy2r_0  SampleTime=-1
  Out : Outport  PortDimensions=10
  wires:
  [ddX2r] -> Mux/9
  [ddY1r] -> Mux/8
  [ddY2r] -> Mux/10
  [ddX1r] -> Mux/7
  [dY2r] -> Sum7/1, Unit Delay 8/1
  [dY1r] -> Unit Delay 7/1, Sum6/1
  Gain 10/1 -> Scope 7/1, [ddY2r]
  Sum7/1 -> Gain 10/1
  Unit Delay 8/1 -> Sum7/2
  Gain 9/1 -> [ddY1r], Scope 6/1
  Sum6/1 -> Gain 9/1
  Unit Delay 7/1 -> Sum6/2
  [dX2r] -> Unit Delay 6/1, Sum5/1
  [dX1r] -> Sum4/1, Unit Delay 5/1
  Gain 8/1 -> [ddX2r], Scope 5/1
  Sum5/1 -> Gain 8/1
  Unit Delay 6/1 -> Sum5/2
  Gain 7/1 -> Scope 4/1, [ddX1r]
  Sum4/1 -> Gain 7/1
  Unit Delay 5/1 -> Sum4/2
  [dO2r] -> Sum3/1, Unit Delay 4/1
  [dO1r] -> Unit Delay 3/1, Sum2/1
  [ddO2r] -> Mux/6
  [ddO1r] -> Mux/3
  [O2r] -> Mux/4
  [dO2r] -> Mux/5
  [dO1r] -> Mux/2
  [O1r] -> Mux/1
  Gain 6/1 -> Scope 3/1, [ddO2r]
  Sum3/1 -> Gain 6/1
  Unit Delay 4/1 -> Sum3/2
  Gain 5/1 -> [ddO1r], Scope 2/1
  Sum2/1 -> Gain 5/1
  Unit Delay 3/1 -> Sum2/2
  Mux/1 -> Out/1
  Gain 4/1 -> [O2r], Scope 9/1, Sum1/1, Unit Delay 2/1
  Trigonometric Function 2/1 -> Interpreted MATLAB Function 2/1, Scope 1/1
  Gain 3/1 -> [dO2r], Scope 13/1
  Sum1/1 -> Gain 3/1
  Unit Delay 2/1 -> Sum1/2
  Interpreted MATLAB Function 2/1 -> Gain 4/1
  [dY2r] -> Trigonometric Function 2/2
  [dX2r] -> Trigonometric Function 2/1
  Gain 2/1 -> Unit Delay 1/1, Sum/1, [O1r], Scope 10/1
  Trigonometric Function 1/1 -> Interpreted MATLAB Function 1/1
  Gain 1/1 -> [dO1r], Scope 14/1
  Sum/1 -> Gain 1/1
  Unit Delay 1/1 -> Sum/2
  Interpreted MATLAB Function 1/1 -> Gain 2/1
  [dY1r] -> Trigonometric Function 1/2
  [dX1r] -> Trigonometric Function 1/1
  Demux2/4 -> [dY2r]
  Demux2/3 -> [dX2r]
  Demux2/2 -> [dY1r]
  Demux2/1 -> [dX1r]
  In/1 -> Demux2/1

== system conSys_2robots_2_vR2014a/Omni Two-Robot ADAMS Model v2015/ADAMS Plant ==
  ADAMS inputs : Inport
  S-Function : S-Function  StopFcn=clear mex  FunctionName=adams_plant  Parameters=exevie,exesol,stat,outfil,nampre,o_rate,nam_in,namout,dft,modsim,modani,dt_out,inicmd,exetyp,comtyp,ada_host, workdir,pin_interp_order,pout_extrap_order,pin_extrap_order,pout_interp_order,simulink_lead_cosim  EnableBusSupport=off
  ADAMS outputs : Outport  InitialOutput=0
  wires:
  S-Function/1 -> ADAMS outputs/1
  ADAMS inputs/1 -> S-Function/1

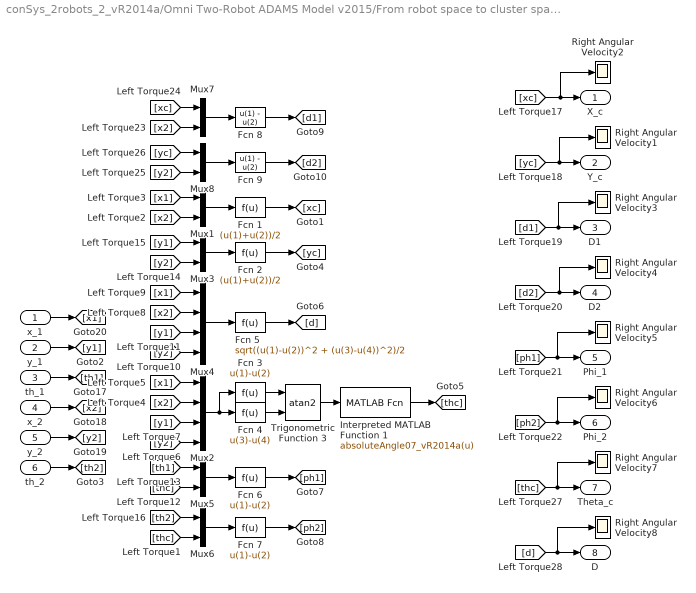
== system conSys_2robots_2_vR2014a/Omni Two-Robot ADAMS Model v2015/From robot space to cluster space 1 ==
  x_1 : Inport
  y_1 : Inport  Port=2
  th_1 : Inport  Port=3
  x_2 : Inport  Port=4
  y_2 : Inport  Port=5
  th_2 : Inport  Port=6
  Fcn 1 : Fcn  Expr=(u(1)+u(2))/2
  Fcn 2 : Fcn  Expr=(u(1)+u(2))/2
  Fcn 3 : Fcn  Expr=u(1)-u(2)
  Fcn 4 : Fcn  Expr=u(3)-u(4)
  Fcn 5 : Fcn  Expr=sqrt((u(1)-u(2))^2 + (u(3)-u(4))^2)/2
  Fcn 6 : Fcn  Expr=u(1)-u(2)
  Fcn 7 : Fcn  Expr=u(1)-u(2)
  Fcn 8 : Fcn  Expr=u(1) - u(2)
  Fcn 9 : Fcn  Expr=u(1) - u(2)
  Interpreted MATLAB Function 1 : MATLABFcn  MATLABFcn=absoluteAngle07_vR2014a(u)  SampleTime=Ts
  Mux{1,3,5..8} (6 alike) : Mux  Inputs=2
  Mux2 : Mux
  Mux4 : Mux
  Right Angular Velocity{1..8} (8 alike) : Scope
      Right Angular Velocity1 settings: YMin=2400  YMax=2600  SaveName=ScopeData38
      Right Angular Velocity2 settings: YMin=2400  YMax=2600  SaveName=ScopeData36
      Right Angular Velocity3 settings: YMin=2400  YMax=2600  SaveName=ScopeData48
      Right Angular Velocity4 settings: YMin=0  YMax=700  SaveName=ScopeData49
      Right Angular Velocity5 settings: YMin=2400  YMax=2600  SaveName=ScopeData50
      Right Angular Velocity6 settings: YMin=2400  YMax=2600  SaveName=ScopeData51
      Right Angular Velocity7 settings: YMin=-10  YMax=10  SaveName=ScopeData80
      Right Angular Velocity8 settings: YMin=1350  YMax=1392.5  SaveName=ScopeData85
  Trigonometric Function 3 : Trigonometry  Operator=atan2
  X_c : Outport
  Y_c : Outport  Port=2
  D1 : Outport  Port=3
  D2 : Outport  Port=4
  Phi_1 : Outport  Port=5
  Phi_2 : Outport  Port=6
  Theta_c : Outport  Port=7
  D : Outport  Port=8
  wires:
  y_2/1 -> [y2]
  x_2/1 -> [x2]
  th_1/1 -> [th1]
  y_1/1 -> [y1]
  x_1/1 -> [x1]
  th_2/1 -> [th2]
  Interpreted MATLAB Function 1/1 -> [thc]
  Trigonometric Function 3/1 -> Interpreted MATLAB Function 1/1
  Mux2/1 -> Fcn 3/1, Fcn 4/1
  Fcn 3/1 -> Trigonometric Function 3/1
  Fcn 4/1 -> Trigonometric Function 3/2
  [x1] -> Mux4/1
  [y2] -> Mux4/4
  [x2] -> Mux4/2
  [y1] -> Mux4/3
  Mux4/1 -> Fcn 5/1
  Fcn 5/1 -> [d]
  [th1] -> Mux5/1
  [thc] -> Mux5/2
  Mux5/1 -> Fcn 6/1
  Fcn 6/1 -> [ph1]
  [xc] -> Right Angular Velocity2/1, X_c/1
  [yc] -> Right Angular Velocity1/1, Y_c/1
  [d1] -> Right Angular Velocity3/1, D1/1
  [d2] -> Right Angular Velocity4/1, D2/1
  [ph1] -> Right Angular Velocity5/1, Phi_1/1
  [ph2] -> Right Angular Velocity6/1, Phi_2/1
  [x1] -> Mux1/1
  [x2] -> Mux1/2
  Mux1/1 -> Fcn 1/1
  Fcn 1/1 -> [xc]
  [y1] -> Mux3/1
  [y2] -> Mux3/2
  Mux3/1 -> Fcn 2/1
  Fcn 2/1 -> [yc]
  [x2] -> Mux2/2
  [x1] -> Mux2/1
  [y2] -> Mux2/4
  [y1] -> Mux2/3
  [th2] -> Mux6/1
  [thc] -> Mux6/2
  Mux6/1 -> Fcn 7/1
  Fcn 7/1 -> [ph2]
  [xc] -> Mux7/1
  [x2] -> Mux7/2
  Mux7/1 -> Fcn 8/1
  Fcn 8/1 -> [d1]
  [yc] -> Mux8/1
  [y2] -> Mux8/2
  Mux8/1 -> Fcn 9/1
  Fcn 9/1 -> [d2]
  [thc] -> Theta_c/1, Right Angular Velocity7/1
  [d] -> Right Angular Velocity8/1, D/1

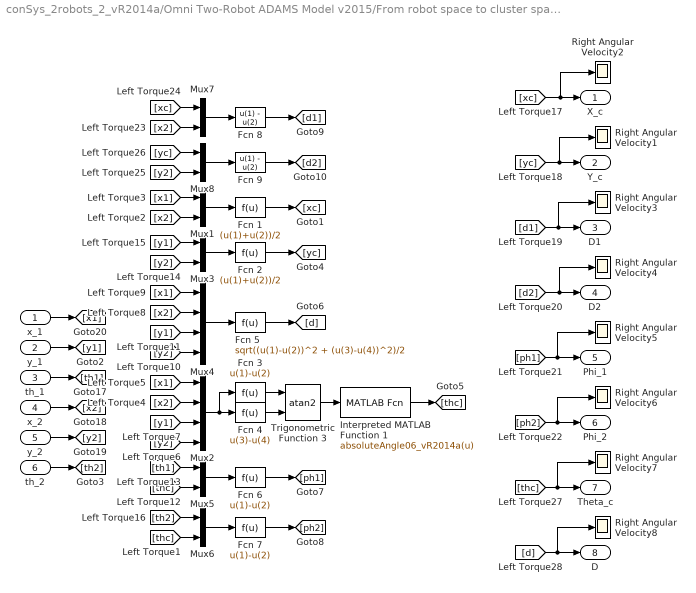
== system conSys_2robots_2_vR2014a/Omni Two-Robot ADAMS Model v2015/From robot space to cluster space 2 ==
  x_1 : Inport
  y_1 : Inport  Port=2
  th_1 : Inport  Port=3
  x_2 : Inport  Port=4
  y_2 : Inport  Port=5
  th_2 : Inport  Port=6
  Fcn 1 : Fcn  Expr=(u(1)+u(2))/2
  Fcn 2 : Fcn  Expr=(u(1)+u(2))/2
  Fcn 3 : Fcn  Expr=u(1)-u(2)
  Fcn 4 : Fcn  Expr=u(3)-u(4)
  Fcn 5 : Fcn  Expr=sqrt((u(1)-u(2))^2 + (u(3)-u(4))^2)/2
  Fcn 6 : Fcn  Expr=u(1)-u(2)
  Fcn 7 : Fcn  Expr=u(1)-u(2)
  Fcn 8 : Fcn  Expr=u(1) - u(2)
  Fcn 9 : Fcn  Expr=u(1) - u(2)
  Interpreted MATLAB Function 1 : MATLABFcn  MATLABFcn=absoluteAngle06_vR2014a(u)  SampleTime=Ts
  Mux{1,3,5..8} (6 alike) : Mux  Inputs=2
  Mux2 : Mux
  Mux4 : Mux
  Right Angular Velocity{1..8} (8 alike) : Scope
      Right Angular Velocity1 settings: YMin=2400  YMax=2600  SaveName=ScopeData38
      Right Angular Velocity2 settings: YMin=2400  YMax=2600  SaveName=ScopeData36
      Right Angular Velocity3 settings: YMin=2400  YMax=2600  SaveName=ScopeData48
      Right Angular Velocity4 settings: YMin=0  YMax=700  SaveName=ScopeData49
      Right Angular Velocity5 settings: YMin=2400  YMax=2600  SaveName=ScopeData50
      Right Angular Velocity6 settings: YMin=2400  YMax=2600  SaveName=ScopeData51
      Right Angular Velocity7 settings: YMin=-10  YMax=10  SaveName=ScopeData80
      Right Angular Velocity8 settings: YMin=1350  YMax=1392.5  SaveName=ScopeData85
  Trigonometric Function 3 : Trigonometry  Operator=atan2
  X_c : Outport
  Y_c : Outport  Port=2
  D1 : Outport  Port=3
  D2 : Outport  Port=4
  Phi_1 : Outport  Port=5
  Phi_2 : Outport  Port=6
  Theta_c : Outport  Port=7
  D : Outport  Port=8
  wires:
  [d] -> D/1, Right Angular Velocity8/1
  [thc] -> Right Angular Velocity7/1, Theta_c/1
  Fcn 9/1 -> [d2]
  Mux8/1 -> Fcn 9/1
  [y2] -> Mux8/2
  [yc] -> Mux8/1
  Fcn 8/1 -> [d1]
  Mux7/1 -> Fcn 8/1
  [x2] -> Mux7/2
  [xc] -> Mux7/1
  Fcn 7/1 -> [ph2]
  Mux6/1 -> Fcn 7/1
  [thc] -> Mux6/2
  [th2] -> Mux6/1
  [y1] -> Mux2/3
  [y2] -> Mux2/4
  [x1] -> Mux2/1
  [x2] -> Mux2/2
  Fcn 2/1 -> [yc]
  Mux3/1 -> Fcn 2/1
  [y2] -> Mux3/2
  [y1] -> Mux3/1
  Fcn 1/1 -> [xc]
  Mux1/1 -> Fcn 1/1
  [x2] -> Mux1/2
  [x1] -> Mux1/1
  [ph2] -> Phi_2/1, Right Angular Velocity6/1
  [ph1] -> Phi_1/1, Right Angular Velocity5/1
  [d2] -> D2/1, Right Angular Velocity4/1
  [d1] -> D1/1, Right Angular Velocity3/1
  [yc] -> Y_c/1, Right Angular Velocity1/1
  [xc] -> X_c/1, Right Angular Velocity2/1
  Fcn 6/1 -> [ph1]
  Mux5/1 -> Fcn 6/1
  [thc] -> Mux5/2
  [th1] -> Mux5/1
  Fcn 5/1 -> [d]
  Mux4/1 -> Fcn 5/1
  [y1] -> Mux4/3
  [x2] -> Mux4/2
  [y2] -> Mux4/4
  [x1] -> Mux4/1
  Fcn 4/1 -> Trigonometric Function 3/2
  Fcn 3/1 -> Trigonometric Function 3/1
  Mux2/1 -> Fcn 4/1, Fcn 3/1
  Trigonometric Function 3/1 -> Interpreted MATLAB Function 1/1
  Interpreted MATLAB Function 1/1 -> [thc]
  th_2/1 -> [th2]
  x_1/1 -> [x1]
  y_1/1 -> [y1]
  th_1/1 -> [th1]
  x_2/1 -> [x2]
  y_2/1 -> [y2]
